simulink model "ejercicio2Comunicaciones"  (R2021a)
settings: Solver=VariableStepAuto  StartTime=0.0  StopTime=0.1  RelTol=1e-3
settings Model: Creator=jmata  LastModifiedBy=jmata

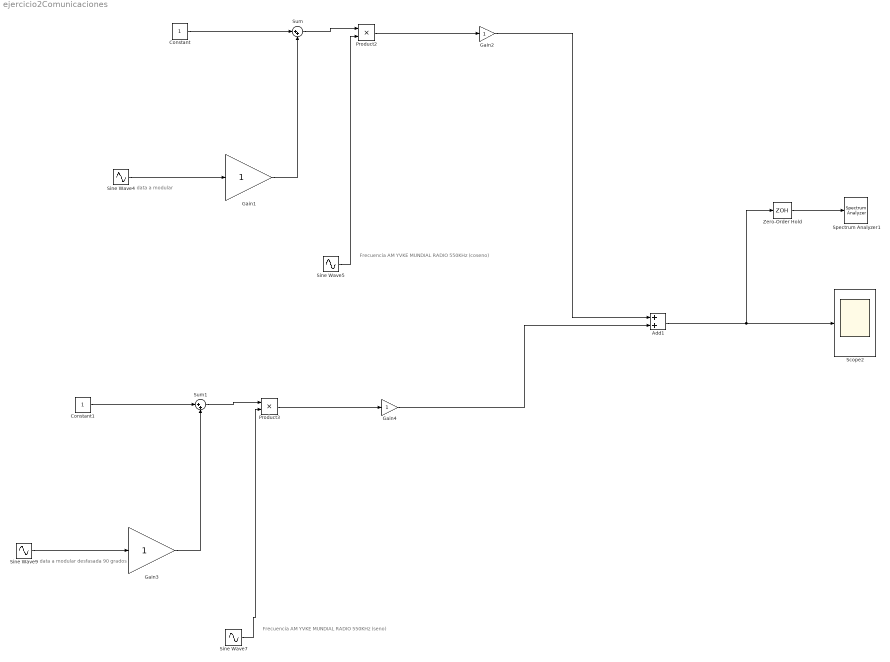
== system ejercicio2Comunicaciones ==
  note: data a modular
  note: Frecuencia AM YVKE MUNDIAL RADIO 550KHz (coseno)
  note: data a modular desfasada 90 grados
  note: Frecuencia AM YVKE MUNDIAL RADIO 550KHz (seno)
  Add1 : Sum
  Constant : Constant
  Constant1 : Constant
  Gain{1..4} (4 alike) : Gain
  Product2 : Product
  Product3 : Product
  Scope2 : Scope
  Sine Wave4 : Sin  Frequency=5e+3 * 2 *pi  SampleTime=0
  Sine Wave5 : Sin  Frequency=550e+3 * 2* pi  Phase=pi/2  SampleTime=0
  Sine Wave7 : Sin  Frequency=550e+3 * 2 * pi  SampleTime=0
  Sine Wave9 : Sin  TimeSource=Use external signal  Frequency=5e+3 * 2 * pi  Phase=pi/2  SampleTime=0
  Spectrum Analyzer1 : SpectrumAnalyzer
  Sum : Sum  Inputs=|++
  Sum1 : Sum  Inputs=|++
  Zero-Order Hold : ZeroOrderHold  SampleTime=-1
  wires:
  Gain1/1 -> Sum/2
  Sine Wave5/1 -> Product2/2
  Product2/1 -> Gain2/1
  Sum/1 -> Product2/1
  Constant/1 -> Sum/1
  Sine Wave4/1 -> Gain1/1
  Gain3/1 -> Sum1/2
  Sine Wave7/1 -> Product3/2
  Product3/1 -> Gain4/1
  Sum1/1 -> Product3/1
  Constant1/1 -> Sum1/1
  Sine Wave9/1 -> Gain3/1
  Gain2/1 -> Add1/1
  Gain4/1 -> Add1/2
  Add1/1 -> Zero-Order Hold/1, Scope2/1
  Zero-Order Hold/1 -> Spectrum Analyzer1/1
